simulink model "EcoSIM3_P2_C2"  (R2014b)
settings: Solver=ode1  SolverMode=SingleTasking  StartTime=0.0  StopTime=inf  FixedStep=0.01  RelTol=1e-3
PostLoadFcn:
  | %, if any(exist('dsrtsu_mdlpostloadfcn', 'file') == [2, 3, 6]), try dsrtsu_mdlpostloadfcn('Execute', bdroot); catch fprintf('Error in PostLoadFcn (dsrtsu_mdlpostloadfcn) for model "%s":\n %s\n', bdroot, lasterr); end, end,
InitFcn:
  | tic
  | %Startup_EcoSIM
values from neighbouring files (symbols this model uses):
  EngPwr = [0 5	10	15	20	25	30	35	40	45	50	55	60	65	70	75	80	85	90	95	100	105	110	115]    [Series_Maps.m]
  EngSpd = [0 477.4645 954.929 1909.858 2864.787 3819.716 4774.645 5729.574 6684.503]    [Series_Maps.m]
  EngTrq = [0	0	0	0	0	0	0	0	0	0	0	0	0	0	0	0	0	0	0	0	0	0	0	0 ... (first row only)    [Series_Maps.m]
  Power = [0 5 10 15 20 25 30]    [Series_Maps.m]
  Torque = [-50,-40,-30,-25,-20,-15,-10,-8,-6,-4,-2,0]    [Series_Maps.m]
undefined symbols (not defined in the file or in its folder): canChannel, Controls, DriveCycles, Driver, EM_EFF_MAP, EM_PwrLoss_MAP, Glbl, Plants, Veh_Dynamics
libraries: canmsglib x100, canlib x87, fl_lib x78, simulink x59, nesl_utility x40, sdl_lib x17, dspsigops x5, dspswit3 x3, dspstat3 x2, commnoisgen2 x1, dspfdesign x1
(part 7 of 15)

== system EcoSIM3_P2_C2/Supervisory Controller/Supervisory_IO/VNT Vector/Electrical Tx ==
  Electrical Tx : Inport
  Bus Creator : BusCreator  Inputs=2
  Bus Selector : BusSelector  OutputSignals=PON,chga_wake
  tag scope: VNT_Electrical_FromMABx=global
  wires:
  Bus Creator/1 -> [VNT_Electrical_FromMABx]  "Supervisory_Electrical_Out"
  Bus Selector/2 -> Bus Creator/2  "<chga_wake>"
  Bus Selector/1 -> Bus Creator/1  "<PON>"
  Electrical Tx/1 -> Bus Selector/1

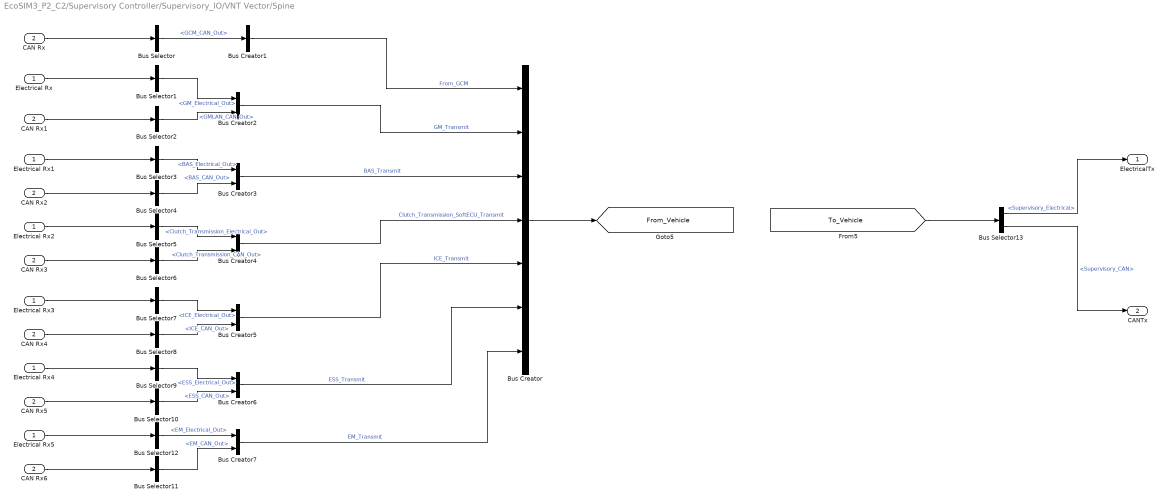
== system EcoSIM3_P2_C2/Supervisory Controller/Supervisory_IO/VNT Vector/Spine ==
  Electrical Rx : Inport
  CAN Rx : Inport  Port=2
  Bus Creator : BusCreator  Inputs=7
  Bus Creator1 : BusCreator  Inputs=1
  Bus Creator{2..7} (6 alike) : BusCreator  Inputs=2
  Bus Selector : BusSelector  OutputSignals=GCM_CAN_Out
  Bus Selector1 : BusSelector  OutputSignals=GM_Electrical_Out
  Bus Selector10 : BusSelector  OutputSignals=ESS_CAN_Out
  Bus Selector11 : BusSelector  OutputSignals=EM_CAN_Out
  Bus Selector12 : BusSelector  OutputSignals=EM_Electrical_Out
  Bus Selector13 : BusSelector  OutputSignals=Supervisory_Electrical,Supervisory_CAN
  Bus Selector2 : BusSelector  OutputSignals=GMLAN_CAN_Out
  Bus Selector3 : BusSelector  OutputSignals=BAS_Electrical_Out
  Bus Selector4 : BusSelector  OutputSignals=BAS_CAN_Out
  Bus Selector5 : BusSelector  OutputSignals=Clutch_Transmission_Electrical_Out
  Bus Selector6 : BusSelector  OutputSignals=Clutch_Transmission_CAN_Out
  Bus Selector7 : BusSelector  OutputSignals=ICE_Electrical_Out
  Bus Selector8 : BusSelector  OutputSignals=ICE_CAN_Out
  Bus Selector9 : BusSelector  OutputSignals=ESS_Electrical_Out
  CAN Rx{1..6} (6 alike) : InportShadow  Port=2
  Electrical Rx{1..5} (5 alike) : InportShadow
  ElectricalTx : Outport
  CANTx : Outport  Port=2
  tag scope: From_Vehicle=global
  wires:
  [To_Vehicle] -> Bus Selector13/1
  Bus Creator/1 -> [From_Vehicle]
  CAN Rx/1 -> Bus Selector/1
  Electrical Rx/1 -> Bus Selector1/1
  Bus Selector/1 -> Bus Creator1/1  "<GCM_CAN_Out>"
  Bus Creator1/1 -> Bus Creator/1  "From_GCM"
  CAN Rx1/1 -> Bus Selector2/1
  Bus Selector1/1 -> Bus Creator2/1  "<GM_Electrical_Out>"
  Bus Selector2/1 -> Bus Creator2/2  "<GMLAN_CAN_Out>"
  Bus Creator2/1 -> Bus Creator/2  "GM_Transmit"
  Electrical Rx1/1 -> Bus Selector3/1
  CAN Rx2/1 -> Bus Selector4/1
  Bus Selector3/1 -> Bus Creator3/1  "<BAS_Electrical_Out>"
  Bus Selector4/1 -> Bus Creator3/2  "<BAS_CAN_Out>"
  Bus Creator3/1 -> Bus Creator/3  "BAS_Transmit"
  Electrical Rx2/1 -> Bus Selector5/1
  CAN Rx3/1 -> Bus Selector6/1
  Bus Selector5/1 -> Bus Creator4/1  "<Clutch_Transmission_Electrical_Out>"
  Bus Selector6/1 -> Bus Creator4/2  "<Clutch_Transmission_CAN_Out>"
  Bus Creator4/1 -> Bus Creator/4  "Clutch_Transmission_SoftECU_Transmit"
  Electrical Rx3/1 -> Bus Selector7/1
  CAN Rx4/1 -> Bus Selector8/1
  Bus Selector7/1 -> Bus Creator5/1  "<ICE_Electrical_Out>"
  Bus Selector8/1 -> Bus Creator5/2  "<ICE_CAN_Out>"
  Bus Creator5/1 -> Bus Creator/5  "ICE_Transmit"
  Electrical Rx4/1 -> Bus Selector9/1
  CAN Rx5/1 -> Bus Selector10/1
  Bus Selector9/1 -> Bus Creator6/1  "<ESS_Electrical_Out>"
  Bus Selector10/1 -> Bus Creator6/2  "<ESS_CAN_Out>"
  Bus Creator6/1 -> Bus Creator/6  "ESS_Transmit"
  Electrical Rx5/1 -> Bus Selector12/1
  CAN Rx6/1 -> Bus Selector11/1
  Bus Selector12/1 -> Bus Creator7/1  "<EM_Electrical_Out>"
  Bus Selector11/1 -> Bus Creator7/2  "<EM_CAN_Out>"
  Bus Creator7/1 -> Bus Creator/7  "EM_Transmit"
  Bus Selector13/1 -> ElectricalTx/1  "<Supervisory_Electrical>"
  Bus Selector13/2 -> CANTx/1  "<Supervisory_CAN>"

== system EcoSIM3_P2_C2/Powertrain/BAS Motor/ Compnent Model/Sensors/Sensor lag ==
  i : Inport
  1st Order LPF of 1ms in Discrete Form : DiscreteTransferFcn  Numerator=[0.6321]  Denominator=[1 -0.3679]
  o : Outport
  wires:
  i/1 -> 1st Order LPF of 1ms in Discrete Form/1
  1st Order LPF of 1ms in Discrete Form/1 -> o/1

== system EcoSIM3_P2_C2/Powertrain/BAS Motor/ Compnent Model/Sensors/Sensor lag1 ==
  i : Inport
  1st Order LPF of 1ms in Discrete Form : DiscreteTransferFcn  Numerator=[0.6321]  Denominator=[1 -0.3679]
  o : Outport
  wires:
  1st Order LPF of 1ms in Discrete Form/1 -> o/1
  i/1 -> 1st Order LPF of 1ms in Discrete Form/1

== system EcoSIM3_P2_C2/Powertrain/BAS Motor/Soft ECU/Algorithm/BAS_Stateflow ==
  note: Notes:
      | 1. Mode Request is similar to Inverter Enable / Disable (to be received from the supervisory controller)
      | 2. Motor Fault is detected by a fault appearing at any of the phases of the motor (other faults can be incorporated in the Fault Subsystem)
  ModeRequest : Inport
  TorqueLimit : Inport  Port=2
  TorqueCommand : Inport  Port=3
  MotorSpeed : Inport  Port=4
  PowerUp : Inport  Port=5
  Speed_cmd : Inport  Port=6
  BAS SoftECU : Stateflow chart  TreatAsAtomicUnit=on
  Bus Creator : BusCreator  Inputs=6
  Bus Selector : BusSelector  OutputSignals=Fault_U,Fault_V,Fault_W
  Bus Selector2 : BusSelector  OutputSignals=Motor_MaxSpeed,POST_Fault
  Constant : Constant  Value=Plants.Belt.GR  SampleTime=0.01
  Contactor_Status : Constant
  Display : Display
  EEPROM Parameters : Subsystem
  Faults : Subsystem
  Gain : Gain  Gain=-1
  Ground : Ground
  Logical Operator : Logic  AllPortsSameDT=off  OutDataTypeStr=boolean
  Multiport Switch : MultiPortSwitch  DataPortOrder=Zero-based contiguous  SampleTime=0.01
  Saturation Dynamic : simulink/Discontinuities/Saturation Dynamic  OutMin=[]  OutMax=[]  OutDataTypeStr=Inherit: Same as second input  OutDataType=fixdt(1, 16)  OutScaling=2^-10  DoSatur=off
  Subsystem : Subsystem
  BAS_Torque_Command_Nm : Outport
  BAS_CAN_Out : Outport  Port=2
  wires:
  EEPROM Parameters/1(EEPROM param) -> Bus Selector2/1
  Bus Selector2/2 -> BAS SoftECU/5(POST_Fault)  "<POST_Fault>"
  Contactor_Status/1 -> Logical Operator/2  "batt_mainc_stat"
  Logical Operator/1 -> BAS SoftECU/1(Power_up)  "Power_up"
  Faults/1(MotorFault) -> BAS SoftECU/2(MotorFault)
  ModeRequest/1 -> Multiport Switch/1, BAS SoftECU/3(ModeRequest)
  Bus Selector2/1 -> BAS SoftECU/4(MotorMaxSpeed)  "<Motor_MaxSpeed>"
  Gain/1 -> Saturation Dynamic/3
  TorqueLimit/1 -> Saturation Dynamic/1, Gain/1
  TorqueCommand/1 -> Saturation Dynamic/2
  MotorSpeed/1 -> Subsystem/2(Speed_feedback_rad_per_s), BAS SoftECU/7(MotorSpeed)
  BAS SoftECU/1(Commanded_Torque) -> Multiport Switch/3, Bus Creator/1
  BAS SoftECU/2(InverterStatusMode) -> Bus Creator/2  "BAS_Status_Mode"
  Bus Creator/1 -> BAS_CAN_Out/1  "BAS CAN Out"
  Faults/2(CAN) -> Bus Selector/1
  Bus Selector/3 -> Bus Creator/6  "<Fault_W>"
  Bus Selector/2 -> Bus Creator/5  "<Fault_V>"
  Bus Selector/1 -> Bus Creator/4  "<Fault_U>"
  BAS SoftECU/3(FaultState) -> Bus Creator/3  "BAS_Fault_Status"
  PowerUp/1 -> Logical Operator/1
  Constant/1 -> BAS SoftECU/8(BeltRatio), Display/1
  Multiport Switch/1 -> BAS_Torque_Command_Nm/1
  Speed_cmd/1 -> BAS SoftECU/9(Speed_Command)
  BAS SoftECU/4(Commanded_Speed) -> Subsystem/1(Speed_command_rpm)
  Ground/1 -> Multiport Switch/2
  Subsystem/1("Torque_command_Nm ") -> Multiport Switch/4
  Saturation Dynamic/1 -> BAS SoftECU/6(Torque_Command)

== system EcoSIM3_P2_C2/Powertrain/Electric Motor / Component Model/Plant/EM_Thermal_Model ==
  note: Instead of a heat source, add convection to the water
  note: A hotspot that will be the thermally weakest point
  note: Assume coolant out temp is same as motor temp
  EM_Power_Loss : Inport
  Conductive Heat Transfer : fl_lib/Thermal/Thermal Elements/Conductive Heat Transfer  area=4 cm^2  thickness=0.1 cm  th_cond=401 W/(m*K)  Q_specify=off  Q_priority=High  Q=0 J/s  T_specify=off  T_priority=High  T=0 K
  Constant1 : Constant  Value=293
  Convection to air : fl_lib/Thermal/Thermal Elements/Convective Heat Transfer  area=1111 cm^2  heat_tr_coeff=10 W/(m^2 * K)  Q_specify=off  Q_priority=High  Q=0 J/s  T_specify=off  T_priority=High  T=0 K
  EM_Over_Temp_Fault : Subsystem
  Gain : Gain  Gain=0.05
  Gain1 : Gain  Gain=0.95
  Heat Dissipated through coolant : Subsystem
  Heat absorbed by coolant : fl_lib/Thermal/Thermal Sources/Ideal Heat Flow Source
  Hotspot Heat : fl_lib/Thermal/Thermal Sources/Ideal Heat Flow Source
  Hotspot Thermal mass : fl_lib/Thermal/Thermal Elements/Thermal Mass  mass=0.1 kg  sp_heat=447 J/kg/K  Q_specify=off  Q_priority=High  Q=0 J/s  T_specify=off  T_priority=High  T=300 K
  Hotspot temp in °C : Scope
      settings: SaveName=ScopeData2
  Ideal Temperature Source : fl_lib/Thermal/Thermal Sources/Ideal Temperature Source
  Memory : Memory  X0=293
  Memory1 : Memory  X0=25
  Motor Heat Loss : fl_lib/Thermal/Thermal Sources/Ideal Heat Flow Source
  Motor Thermal Mass : fl_lib/Thermal/Thermal Elements/Thermal Mass  mass=35 kg  sp_heat=447 J/kg/K  Q_specify=off  Q_priority=High  Q=0 J/s  T_specify=off  T_priority=High  T=300 K
  Simulink-PS Converter : nesl_utility/Simulink-PS Converter  PhysicalDomain=network_engine_domain  SubClassName=ps_input  LeftPortType=input  RightPortType=output  PseudoPeriodic=off  Frequencies=[]  NoiseDistribution=none  NoiseParameters=[]  Unit=J/s  AffineConversion=off  InputFiltering=off  SimscapeFilterOrder=1  InputFilterTimeConstant=0.001  UdotUserProvided=1
  Simulink-PS Converter1 : nesl_utility/Simulink-PS Converter  PhysicalDomain=network_engine_domain  SubClassName=ps_input  LeftPortType=input  RightPortType=output  PseudoPeriodic=off  Frequencies=[]  NoiseDistribution=none  NoiseParameters=[]  Unit=J/s  AffineConversion=off  InputFiltering=off  SimscapeFilterOrder=1  InputFilterTimeConstant=0.001  UdotUserProvided=1
  Simulink-PS Converter2 : nesl_utility/Simulink-PS Converter  PhysicalDomain=network_engine_domain  SubClassName=ps_input  LeftPortType=input  RightPortType=output  PseudoPeriodic=off  Frequencies=[]  NoiseDistribution=none  NoiseParameters=[]  Unit=K  AffineConversion=off  InputFiltering=off  SimscapeFilterOrder=1  InputFilterTimeConstant=0.001  UdotUserProvided=1
  Solver Configuration : nesl_utility/Solver Configuration  PhysicalDomain=network_engine_domain  SubClassName=solver  LeftPortType=input  RightPortType=generic  Accelerate=off  Tones=[]  Harmonics=[]  SimulateNoise=off  Profile=off  UseLocalSampling=off  EnableSwitchedLinearOptims=on  FrequencyDomain=off  UseCCode=off  RelTol=0.001  AbsTol=1e-06  MinStep=1e-09  ToWorkspace=off  DoDC=off  ResidualTolerance=1e-09  UseLocalSolver=on  LocalSolverChoice=NE_BACKWARD_EULER_ADVANCER  LocalSolverSampleTime=0.01  DoFixedCost=off  MaxNonlinIter=3  MaxModeIter=2  LinearAlgebra=Sparse  DelaysMemoryBudget=1024  AutomaticFiltering=on  FilteringTimeConstant=0.001
  Temp Hotspot : Subsystem
  Temp Motor : Subsystem
  Thermal Reference{,2..4} (4 alike) : fl_lib/Thermal/Thermal Elements/Thermal Reference
  Out1 : Outport
  wires:
  Constant1/1 -> Simulink-PS Converter2/1
  Temp Hotspot/1(Temp C) -> Hotspot temp in °C/1  "EM_hotspot_Temperature_degC"
  Temp Motor/1(Temp K) -> Memory/1
  EM_Over_Temp_Fault/1(Out1) -> Out1/1  "EM_Temperature_degC"
  Memory/1 -> Heat Dissipated through coolant/1(Coolant Out Temp)
  EM_Power_Loss/1 -> Gain/1, Gain1/1  "EM_Power_loss_W"
  Gain/1 -> Simulink-PS Converter/1
  Gain1/1 -> Simulink-PS Converter1/1
  Temp Motor/2(Temp C) -> Memory1/1  "EM_Temperature_degC"
  Memory1/1 -> EM_Over_Temp_Fault/1(In1)  "EM_Temperature_degC"
  connections:
  Simulink-PS Converter2/RConn1 -- Ideal Temperature Source/RConn1
  Heat Dissipated through coolant/RConn1 -- Heat absorbed by coolant/RConn1
  Convection to air/RConn1 -- Ideal Temperature Source/LConn1
  Thermal Reference4/LConn1 -- Hotspot Heat/RConn2
  Simulink-PS Converter1/RConn1 -- Hotspot Heat/RConn1
  Thermal Reference/LConn1 -- Motor Heat Loss/RConn2
  Thermal Reference2/LConn1 -- Ideal Temperature Source/RConn2
  Thermal Reference3/LConn1 -- Heat absorbed by coolant/RConn2
  Motor Heat Loss/RConn1 -- Simulink-PS Converter/RConn1 -- Solver Configuration/RConn1
  Convection to air/LConn1 -- Temp Motor/LConn1 -- Conductive Heat Transfer/RConn1 -- Motor Thermal Mass/LConn1 -- Heat absorbed by coolant/LConn1 -- Motor Heat Loss/LConn1
  Conductive Heat Transfer/LConn1 -- Hotspot Thermal mass/LConn1 -- Temp Hotspot/LConn1 -- Hotspot Heat/LConn1

== system EcoSIM3_P2_C2/Powertrain/Electric Motor / Component Model/Sensors/Fault Insertation ==
  In1 : Inport
  Additional_Torque_Nm_Default : Constant  Value=0
  Gain : Gain  Gain=.3
  Ideal Torque Source1 : fl_lib/Mechanical/Mechanical Sources/Ideal Torque Source
  Mechanical Rotational Reference2 : fl_lib/Mechanical/Rotational Elements/Mechanical Rotational Reference
  OverTorque_Trigger : Switch  Criteria=u2 > Threshold  Threshold=0.5
  Simulink-PS Converter1 : nesl_utility/Simulink-PS Converter  PhysicalDomain=network_engine_domain  SubClassName=ps_input  LeftPortType=input  RightPortType=output  PseudoPeriodic=off  Frequencies=[]  NoiseDistribution=none  NoiseParameters=[]  Unit=1  AffineConversion=off  InputFiltering=off  SimscapeFilterOrder=1  InputFilterTimeConstant=0.001  UdotUserProvided=1
  Conn1 : PMIOPort  Port=1  Side=Right
  wires:
  [EM_OverTorque_Trigger] -> OverTorque_Trigger/2
  Additional_Torque_Nm_Default/1 -> OverTorque_Trigger/3
  OverTorque_Trigger/1 -> Simulink-PS Converter1/1
  In1/1 -> Gain/1
  Gain/1 -> OverTorque_Trigger/1
  connections:
  Simulink-PS Converter1/RConn1 -- Ideal Torque Source1/RConn1
  Ideal Torque Source1/RConn2 -- Mechanical Rotational Reference2/LConn1
  Ideal Torque Source1/LConn1 -- Conn1/RConn1

== system EcoSIM3_P2_C2/Powertrain/Electric Motor / Component Model/Sensors/Sensor lag ==
  i : Inport
  1st Order LPF of 1ms in Discrete Form : DiscreteTransferFcn  Numerator=[0.6321]  Denominator=[1 -0.3679]
  o : Outport
  wires:
  i/1 -> 1st Order LPF of 1ms in Discrete Form/1
  1st Order LPF of 1ms in Discrete Form/1 -> o/1

== system EcoSIM3_P2_C2/Powertrain/Electric Motor / Component Model/Sensors/Sensor lag1 ==
  i : Inport
  1st Order LPF of 1ms in Discrete Form : DiscreteTransferFcn  Numerator=[0.6321]  Denominator=[1 -0.3679]
  o : Outport
  wires:
  i/1 -> 1st Order LPF of 1ms in Discrete Form/1
  1st Order LPF of 1ms in Discrete Form/1 -> o/1

== system EcoSIM3_P2_C2/Powertrain/Electric Motor / Component Model/Sensors/Sensors ==
  note: Sensor Model: Place where we add Corrupter
  Bus Creator : BusCreator  Inputs=2
  Ideal Rotational Motion Sensor : fl_lib/Mechanical/Mechanical Sensors/Ideal Rotational Motion Sensor  offset=0 rad
  Ideal Torque Sensor : fl_lib/Mechanical/Mechanical Sensors/Ideal Torque Sensor
  Mechanical Rotational Reference1 : fl_lib/Mechanical/Rotational Elements/Mechanical Rotational Reference
  PS-Simulink Converter : nesl_utility/PS-Simulink Converter  PhysicalDomain=network_engine_domain  SubClassName=ps_output  LeftPortType=input  RightPortType=output  PseudoPeriodic=off  Frequencies=[]  Unit=1  AffineConversion=off
  PS-Simulink Converter1 : nesl_utility/PS-Simulink Converter  PhysicalDomain=network_engine_domain  SubClassName=ps_output  LeftPortType=input  RightPortType=output  PseudoPeriodic=off  Frequencies=[]  Unit=1  AffineConversion=off
  Sensor lag : Subsystem
  Sensor lag1 : Subsystem
  Shaft : PMIOPort  Port=1  Side=Left
  To_Plants : PMIOPort  Port=2  Side=Right
  EM_Shaft_out : Outport
  wires:
  Sensor lag/1(o) -> Bus Creator/1  "EM_Speed_produced_rad_per_s"
  Sensor lag1/1(o) -> Bus Creator/2  "EM_Torque_Produced_Nm"
  Bus Creator/1 -> EM_Shaft_out/1  "EM_Shaft"
  PS-Simulink Converter/1 -> Sensor lag/1(i)  "EM_Speed_produced_rad_per_s"
  PS-Simulink Converter1/1 -> Sensor lag1/1(i)  "EM_Torque_Produced_Nm"
  connections:
  Ideal Torque Sensor/LConn1 -- Shaft/RConn1 -- Ideal Rotational Motion Sensor/LConn1
  Ideal Rotational Motion Sensor/RConn1 -- Mechanical Rotational Reference1/LConn1
  PS-Simulink Converter/LConn1 -- Ideal Rotational Motion Sensor/RConn2
  PS-Simulink Converter1/LConn1 -- Ideal Torque Sensor/RConn2
  Ideal Torque Sensor/RConn1 -- To_Plants/RConn1

== system EcoSIM3_P2_C2/Powertrain/Electric Motor /Soft ECU/Algorithm/Normal Operation ==
  note: These signals are supposed to be
      |  coming in through CAN
  SignalIn : Inport
  Ignition Switch : Inport  Port=2
  FaultTrigger : Inport  Port=3
  Sensors : Inport  Port=4
  Enable : EnablePort  StatesWhenEnabling=reset
  Bus Selector : BusSelector  OutputSignals=Motor_MaxSpeed
  Bus Selector1 : BusSelector  OutputSignals=EM_CAN_Messages.EM_CAN.M192_Command_Message.Rotation_Direction,EM_CAN_Messages.EM_CAN.M192_Command_Message.Torque_Command,ESS_CAN_Out.BCM_Status.bcm_mainc_stat,EM_CAN_Messages.EM_CAN.M192_Command_Message.Inverter_Enable
  Bus Selector2 : BusSelector  OutputSignals=Motor_Speed,InternalMotorError
  Bus Selector3 : BusSelector  OutputSignals=GMLAN_CAN_Out.PPEI_Platform_General_Status.SysPwrMd
  Bus Selector4 : BusSelector  OutputSignals=EM_torque_cmd_value,EM_torque_cmd_trigger
  EEPROM Parameters1 : Subsystem
  Normal_Operation : Stateflow chart  TreatAsAtomicUnit=on
  Switch : Switch  Criteria=u2 > Threshold  Threshold=0.5
  Commanded_Torque : Outport
  RUN_Fault : Outport  Port=2
  ShutdownRequest : Outport  Port=3  OutputWhenDisabled=reset  InitialOutput=0
  wires:
  Normal_Operation/2(RUN_Fault) -> RUN_Fault/1
  Bus Selector1/1 -> Normal_Operation/3(Rotation_Direction)  "<Rotation_Direction>"
  Bus Selector1/2 -> Normal_Operation/4(Torque_Command)  "<Torque_Command>"
  SignalIn/1 -> Bus Selector1/1
  Bus Selector/1 -> Normal_Operation/8(Motor_MaxSpeed)  "<Motor_MaxSpeed>"
  Sensors/1 -> Bus Selector2/1
  Bus Selector2/1 -> Normal_Operation/1(Motor_Speed)  "<Motor_Speed>"
  Bus Selector2/2 -> Normal_Operation/2(InternalMotorError)  "<InternalMotorError>"
  Normal_Operation/1(Commanded_Torque) -> Switch/3
  EEPROM Parameters1/1(EEPROM param) -> Bus Selector/1
  Bus Selector1/3 -> Normal_Operation/5(batt_mainc_stat)  "<bcm_mainc_stat>"
  Ignition Switch/1 -> Bus Selector3/1
  Bus Selector3/1 -> Normal_Operation/7(IgnitionKeySw)  "<SysPwrMd>"
  Normal_Operation/3(ShutdownRequest) -> ShutdownRequest/1
  Bus Selector1/4 -> Normal_Operation/6(Inverter_Enable)  "<Inverter_Enable>"
  Switch/1 -> Commanded_Torque/1  "Commanded_Torque"
  FaultTrigger/1 -> Bus Selector4/1
  Bus Selector4/2 -> Switch/2  "<EM_torque_cmd_trigger>"
  Bus Selector4/1 -> Switch/1  "<EM_torque_cmd_value>"

== system EcoSIM3_P2_C2/Powertrain/Electric Motor /Soft ECU/Algorithm/Rinehart Documentation ==

== system EcoSIM3_P2_C2/Powertrain/Electric Motor /Soft ECU/Algorithm/Startup_Shutdown ==
  SignalIn : Inport
  Ignition Switch : Inport  Port=2
  RUN_Fault : Inport  Port=3
  ShutDownRequest : Inport  Port=4
  Bus Selector : BusSelector  OutputSignals=EM_CAN_Messages.EM_Electrical.EM_Powerup,EM_Sensors.InternalMotorError,ESS_CAN_Out.BCM_Status.bcm_mainc_stat,EM_CAN_Messages.EM_CAN.M192_Command_Message.Inverter_Enable
  Bus Selector1 : BusSelector  OutputSignals=KeySwMode,POST_Fault
  Bus Selector2 : BusSelector  OutputSignals=GMLAN_CAN_Out.PPEI_Platform_General_Status.SysPwrMd
  Bus Selector3 : BusSelector  Commented=on  OutputSignals=EM_Powerup
  Display : Display
  Display1 : Display
  EEPROM Parameters : Subsystem
  From : From  Commented=on  GotoTag=Powerups  TagVisibility=global
  Memory : Memory
  Startup-Shutdown : Stateflow chart  TreatAsAtomicUnit=on
  VSM_Mode : Outport
  Inverter_Enable_Lockout : Outport  Port=2
  Inverter_Status : Outport  Port=3
  POST_Fault : Outport  Port=4
  wires:
  Startup-Shutdown/1(VSM_Mode) -> VSM_Mode/1
  Startup-Shutdown/2(Inverter_Enable_Lockout) -> Display1/1, Inverter_Enable_Lockout/1  "Inverter_Enable_Lockout"
  RUN_Fault/1 -> Startup-Shutdown/6(RUN_Fault)
  ShutDownRequest/1 -> Memory/1
  Bus Selector/2 -> Startup-Shutdown/2(InternalMotorError)  "<InternalMotorError>"
  SignalIn/1 -> Bus Selector/1
  EEPROM Parameters/1(EEPROM param) -> Bus Selector1/1
  Bus Selector1/1 -> Startup-Shutdown/8(KeySwMode)  "<KeySwMode>"
  Bus Selector1/2 -> POST_Fault/1, Startup-Shutdown/9(POST_Fault)  "<POST_Fault>"
  Bus Selector/3 -> Startup-Shutdown/3(batt_mainc_stat)  "<bcm_mainc_stat>"
  Bus Selector/4 -> Display/1, Startup-Shutdown/4(Inverter_Enable)  "<Inverter_Enable>"
  Startup-Shutdown/3(Inverter_Status) -> Inverter_Status/1
  Ignition Switch/1 -> Bus Selector2/1
  Bus Selector2/1 -> Startup-Shutdown/5(IgnitionKeySw)  "<SysPwrMd>"
  Memory/1 -> Startup-Shutdown/7(ShutdownRequest)
  Bus Selector/1 -> Startup-Shutdown/1(Power_up)  "<EM_Powerup>"

== system EcoSIM3_P2_C2/Powertrain/Electric Motor /Soft ECU/Algorithm/Temperature Values Dummy ==
  FromPlant : Inport
  Bus Creator : BusCreator  Inputs=6
  Control_Board_Temperature : Constant  Value=25
  ESS_Over_Temp_Fault : Subsystem
  Gain : Gain
  Gate_Driver_Board : Constant  Value=25
  Module_A : Constant  Value=25
  Module_B : Constant  Value=25
  Module_C : Constant  Value=25
  TempValues : Outport
  wires:
  ESS_Over_Temp_Fault/1(Out1) -> Bus Creator/1  "Module_A"
  Bus Creator/1 -> TempValues/1
  Module_B/1 -> Bus Creator/2  "Module_B"
  Module_C/1 -> Bus Creator/3  "Module_C"
  Gate_Driver_Board/1 -> Bus Creator/4  "Gate_Driver_Board"
  Control_Board_Temperature/1 -> Bus Creator/5  "Control_Board_Temperature"
  FromPlant/1 -> Gain/1
  Gain/1 -> Bus Creator/6  "Motor_Temperature"
  Module_A/1 -> ESS_Over_Temp_Fault/1(In1)

== system EcoSIM3_P2_C2/Powertrain/Electrical Storage System/ ESS Model/Plant/Electrical Plant Model ==
  P_in [W] : Inport
  Batt_Temp [C] : Inport  Port=2
  Current Calculation (Per Cell) : Subsystem
  Heat Calculation : Subsystem
  Memory1 : Memory  X0=300
  OCV Estimation : Subsystem
  "Resistance Estimation (Per Cell) " : Subsystem
  SOC Estimation (Per Cell) : Subsystem
  Terminal Voltage Calculation : Subsystem
  Batt_Current [A] : Outport
  Batt_SOC [%] : Outport  Port=2
  Batt_volt [V] : Outport  Port=3
  Batt_Heat [W] : Outport  Port=4
  Batt_volt_1 [V] : Outport  Port=5
  wires:
  P_in [W]/1 -> SOC Estimation (Per Cell)/1(P_in [W]), Current Calculation (Per Cell)/1(P_in [W])
  Terminal Voltage Calculation/1(Batt_Volt [V]) -> Batt_volt [V]/1, Memory1/1
  Current Calculation (Per Cell)/2(Cell_Current [A]) -> "Resistance Estimation (Per Cell) "/1(Cell_Current [A]), Heat Calculation/1(Cell_Current [A]), Terminal Voltage Calculation/3(Cell_Current [A]), OCV Estimation/2(Cell_Current [A])
  SOC Estimation (Per Cell)/1(SOC [%]) -> "Resistance Estimation (Per Cell) "/3(SOC [%]), Batt_SOC [%]/1, OCV Estimation/1(SOC [%])
  OCV Estimation/1(OCV [V]) -> Terminal Voltage Calculation/2(OCV [V])
  Current Calculation (Per Cell)/1(Batt_Current [A]) -> Batt_Current [A]/1
  Heat Calculation/1(Batt_Heat [W]) -> Batt_Heat [W]/1
  "Resistance Estimation (Per Cell) "/1(R_cell [Ohms]) -> Terminal Voltage Calculation/1(R_cell [Ohms]), Heat Calculation/2(R_cell [Ohms])
  Memory1/1 -> Batt_volt_1 [V]/1, Current Calculation (Per Cell)/2(Batt_volt [V])
  Batt_Temp [C]/1 -> "Resistance Estimation (Per Cell) "/2(Cell_Temp [C])

== system EcoSIM3_P2_C2/Powertrain/Electrical Storage System/ ESS Model/Plant/Power Calculation ==
  Input_Crnt [A] : Inport
  Batt_volt_1 [V] : Inport  Port=2
  Component_Power_Watts : Inport  Port=3
  Avg Power Calculation : Subsystem
  Integrator1 : Integrator
  P_in [W] : Outport
  Batt_Electrical_Energy : Outport  Port=2
  Batt_Electrical_Energy_Net : Outport  Port=3
  wires:
  Avg Power Calculation/1(P_in [W]) -> Batt_Electrical_Energy/1, Integrator1/1, P_in [W]/1  "Batt_Electrical_Energy"
  Input_Crnt [A]/1 -> Avg Power Calculation/1(Input_Crnt [A])
  Batt_volt_1 [V]/1 -> Avg Power Calculation/2(Batt_volt_1 [V])
  Integrator1/1 -> Batt_Electrical_Energy_Net/1  "Batt_Electrical_Energy_Net"
  Component_Power_Watts/1 -> Avg Power Calculation/3(Component_Power_Watts)

== system EcoSIM3_P2_C2/Powertrain/Electrical Storage System/ ESS Model/Plant/Thermal Model ==
  note: 1/7
  note: 273+30
  Batt_Heat [W] : Inport
  Constant : Constant  Value=Plants.ESS.Mdl.Plant.Therm_Mdl.T_amb
  Constant5 : Constant  Value=273
  EM_Over_Temp_Fault : Subsystem
  Fcn2 : Fcn  Expr=u/19395
  Fcn3 : Fcn  Expr=u/(193.52*19395)
  Heat input for pack1 : Gain  Gain=1/Plants.ESS.Mdl.Plant.Therm_Mdl.M
  Integrator : Integrator  InitialConditionSource=external
  Subtract : Sum  Inputs=+-
  Subtract3 : Sum  Inputs=-+
  Subtract4 : Sum  Inputs=+-
  T_ambient : Constant  Value=Plants.ESS.Mdl.Plant.Therm_Mdl.T_amb
  Batt_Temp [C] : Outport
  wires:
  Batt_Heat [W]/1 -> Heat input for pack1/1
  Integrator/1 -> Subtract/1, Subtract4/1  "T_B"
  Subtract3/1 -> Integrator/1  "T_B_dot"
  T_ambient/1 -> Subtract/2
  Subtract/1 -> Fcn3/1
  Fcn2/1 -> Subtract3/2
  Constant/1 -> Integrator/2
  Constant5/1 -> Subtract4/2
  EM_Over_Temp_Fault/1(Out1) -> Batt_Temp [C]/1  "Batt_Temp_C"
  Heat input for pack1/1 -> Fcn2/1
  Fcn3/1 -> Subtract3/1
  Subtract4/1 -> EM_Over_Temp_Fault/1(In1)  "Batt_Temp_C"

== system EcoSIM3_P2_C2/Powertrain/Electrical Storage System/Soft ECU/Algorithm/A123 Documentation ==

== system EcoSIM3_P2_C2/Powertrain/Electrical Storage System/Soft ECU/Algorithm/A123 soft ECU ==
  From ECUs : Inport
  A123 BMS : Stateflow chart  TreatAsAtomicUnit=on
  Bus Creator : BusCreator  Inputs=11
  Bus Selector : BusSelector  OutputSignals=BMS_Powerup,hsc_bcm_enable,hsc_bcm_mainc_close,bcm_cell_tmax,hsc_bcm_epo,hsc_bcm_leakage_ena,chga_wake
  Bus Selector1 : BusSelector  OutputSignals=GMLAN_CAN_Out.PPEI_Platform_General_Status.SysPwrMd
  Bus Selector2 : BusSelector  OutputSignals=bcm_alarm_type,bcm_alarm_trigger
  Constant : Constant  Value=65
  Constant1 : Constant  Value=-40
  Constant2 : Constant  Value=0
  Memory{,1..10} (11 alike) : Memory
  Switch : Switch  Criteria=u2 > Threshold  Threshold=0.5
  To ECUs : Outport
  wires:
  From ECUs/1 -> Bus Selector/1
  Bus Selector/2 -> A123 BMS/2(hsc_bcm_enable)  "<hsc_bcm_enable>"
  Bus Selector/3 -> A123 BMS/3(hsc_bcm_mainc_close)  "<hsc_bcm_mainc_close>"
  Constant/1 -> A123 BMS/5(bcm_cell_tmax)
  Constant1/1 -> A123 BMS/6(bcm_cell_tmin)
  Bus Selector/5 -> A123 BMS/7(hsc_bcm_epo)  "<hsc_bcm_epo>"
  Memory3/1 -> Bus Creator/4  "bcm_chgc_stat"
  Memory1/1 -> Bus Creator/3  "bcm_mainc_stat"
  Memory2/1 -> Bus Creator/5  "bcm_cpwr_cmd"
  Memory4/1 -> Bus Creator/2  "bcm_hvil_mon"
  Memory5/1 -> Bus Creator/6  "bcm_cpwr_mon"
  Memory/1 -> Bus Creator/1  "bcm_ready"
  Memory6/1 -> Bus Creator/7  "bcm_epo"
  Bus Creator/1 -> To ECUs/1
  Bus Selector/6 -> A123 BMS/8(hsc_bcm_leakage_ena)  "<hsc_bcm_leakage_ena>"
  [GM_Transmit] -> Bus Selector1/1
  Bus Selector1/1 -> A123 BMS/10(Veh_Start)  "<SysPwrMd>"
  A123 BMS/1(bcm_ready) -> Memory/1  "bcm_ready"
  A123 BMS/4(bcm_chgc_stat) -> Memory3/1  "bcm_chgc_stat"
  A123 BMS/7(bcm_epo) -> Memory6/1  "bcm_epo"
  A123 BMS/6(bcm_cpwr_mon) -> Memory5/1  "bcm_cpwr_mon"
  A123 BMS/5(bcm_cpwr_cmd) -> Memory2/1  "bcm_cpwr_cmd"
  A123 BMS/3(bcm_mainc_stat) -> Memory1/1  "bcm_mainc_stat"
  A123 BMS/2(bcm_hvil_mon) -> Memory4/1  "bcm_hvil_mon"
  Memory7/1 -> Bus Creator/8  "bcm_veh_mon"
  A123 BMS/8(bcm_veh_mon) -> Memory7/1
  Bus Selector/1 -> A123 BMS/1(PowerUp)  "<BMS_Powerup>"
  A123 BMS/9(chga_ena) -> Memory8/1
  Memory8/1 -> Bus Creator/9  "chga_ena"
  Bus Selector/7 -> A123 BMS/9(chga_wake)  "<chga_wake>"
  A123 BMS/10(bcm_on_plug) -> Memory9/1
  Memory9/1 -> Bus Creator/10  "bcm_on_plug"
  Bus Selector/4 -> A123 BMS/4(bcm_cell_temp)  "<bcm_cell_tmax>"
  Constant2/1 -> Switch/3
  Memory10/1 -> Bus Creator/11  "bcm_alarm"
  [BCM_Alarm_Trigger] -> Bus Selector2/1
  Bus Selector2/1 -> Switch/1  "<bcm_alarm_type>"
  Bus Selector2/2 -> Switch/2  "<bcm_alarm_trigger>"
  Switch/1 -> Memory10/1

== system EcoSIM3_P2_C2/Powertrain/Engine/ Component Model/Sensors/Sensor lag ==
  i : Inport
  1st Order LPF of 1ms in Discrete Form : DiscreteTransferFcn  Numerator=[0.6321]  Denominator=[1 -0.3679]
  o : Outport
  wires:
  i/1 -> 1st Order LPF of 1ms in Discrete Form/1
  1st Order LPF of 1ms in Discrete Form/1 -> o/1

== system EcoSIM3_P2_C2/Powertrain/Engine/ Component Model/Sensors/Sensor lag1 ==
  i : Inport
  1st Order LPF of 1ms in Discrete Form : DiscreteTransferFcn  Numerator=[0.6321]  Denominator=[1 -0.3679]
  o : Outport
  wires:
  i/1 -> 1st Order LPF of 1ms in Discrete Form/1
  1st Order LPF of 1ms in Discrete Form/1 -> o/1

== system EcoSIM3_P2_C2/Powertrain/Soft_ECUs_IO/From_Goto/Subsystem1/BAS_Relay ==
  In1 : Inport
  Constant6 : Constant
  Constant7 : Constant  Value=0
  Relay3 : Switch  Criteria=u2 > Threshold  Threshold=0.5
  Out1 : Outport
  wires:
  Constant6/1 -> Relay3/1
  Relay3/1 -> Out1/1  "BAS_Powerup"
  Constant7/1 -> Relay3/3
  In1/1 -> Relay3/2

== system EcoSIM3_P2_C2/Powertrain/Soft_ECUs_IO/From_Goto/Subsystem1/EM_Relay ==
  In1 : Inport
  Constant2 : Constant
  Constant3 : Constant  Value=0
  Relay1 : Switch  Criteria=u2 > Threshold  Threshold=0.5
  Out1 : Outport
  wires:
  Relay1/1 -> Out1/1  "EM_Powerup"
  Constant2/1 -> Relay1/1
  Constant3/1 -> Relay1/3
  In1/1 -> Relay1/2

== system EcoSIM3_P2_C2/Powertrain/Soft_ECUs_IO/From_Goto/Subsystem1/Engine_Relay ==
  In1 : Inport
  Constant4 : Constant
  Constant5 : Constant  Value=0
  Relay2 : Switch  Criteria=u2 > Threshold  Threshold=0.5
  Out1 : Outport
  wires:
  Relay2/1 -> Out1/1  "ICE_Powerup"
  Constant5/1 -> Relay2/3
  Constant4/1 -> Relay2/1
  In1/1 -> Relay2/2

== system EcoSIM3_P2_C2/Powertrain/Soft_ECUs_IO/VNT Kvaser/CANRx/BAS Receive ==
  Bus Creator12 : BusCreator  Inputs=1
  Bus Creator2 : BusCreator  Inputs=2
  CAN Receive : canlib/CAN Receive  BlockHandle=2745.0026  DeviceMenu=Kvaser Virtual 1 (Channel 1)  Device=Kvaser Virtual 1 (Channel 1)  ObjConstructor=canChannel('Kvaser', 'Virtual 1', 1)  EnableStandardIDsFilter=off  StandardIDs=102  EnableExtendedIDsFilter=off  ExtendedIDs=0  SampleTime=0.01  MsgsPerTimestep=1  StdIDsCombo=Allow only  ExtIDsCombo=Block all  InternalFilterUpdateStatus=on
  CAN Unpack : canmsglib/CAN Unpack  CANdbFile=C:\Users\EcoCAR_HIL\Documents\Khanna\EcoSIM3_P1_0_PHEV_TCU\Final_DBC\Engine_Transmission_BAS.dbc  MsgList=ECO_BAS_Receive_MSG102  MsgName=ECO_BAS_Receive_MSG102  MsgIDType=Standard (11-bit identifier)  MsgIdentifier=102  MsgLength=2  SignalInfo=BAS_Mode_Request$8$1$2$2$1$0$1$0$0$1$#BAS_Torque_Request_Nm$9$15$2$1$1$0$1.000000e-02$0$-1.638400e+02$1.638300e+02$#  NSignals=2  IDPort=off  TimestampPort=off  ErrorPort=off  RemotePort=off  LengthPort=off  StatusPort=off  StartBits=str2num('[int32(8);int32(9)]')  SignalSizes=str2num('[int32(1);int32(15)]')  ByteOrders=str2num('[int32(2);int32(2)]')  DataTypes=str2num('[int32(2);int32(1)]')  MultiplexTypes=str2num('[int32(1);int32(1)]')  MultiplexValues=str2num('[double(0);double(0)]')  Factors=str2num('[double(1);double(1.000000e-02)]')  Offsets=str2num('[double(0);double(0)]')  Minimums=str2num('[double(0);double(-1.638400e+02)]')  Maximums=str2num('[double(1);double(1.638300e+02)]')
      settings: DataFormat=CANdb specified signals
  Terminator6 : Terminator
  BAS_CAN : Outport
  wires:
  Bus Creator12/1 -> BAS_CAN/1  "BAS_CAN"
  Bus Creator2/1 -> Bus Creator12/1  "SetValues"
  CAN Receive/1 -> Terminator6/1
  CAN Unpack/1 -> Bus Creator2/1  "BAS_Mode_Request"
  CAN Unpack/2 -> Bus Creator2/2  "BAS_Torque_Request_Nm"
  CAN Receive/2 -> CAN Unpack/1

== system EcoSIM3_P2_C2/Powertrain/Soft_ECUs_IO/VNT Kvaser/CANRx/Brusa Receive ==
  Bus Creator4 : BusCreator  Inputs=2
  Ground : Ground
  Ground1 : Ground
  Brusa CAN : Outport
  wires:
  Bus Creator4/1 -> Brusa CAN/1  "Brusa_CAN"
  Ground/1 -> Bus Creator4/1  "Dummy1"
  Ground1/1 -> Bus Creator4/2  "Dummy2"

== system EcoSIM3_P2_C2/Powertrain/Soft_ECUs_IO/VNT Kvaser/CANRx/EM Receive ==
  Bus Creator : BusCreator  Inputs=1
  Bus Creator1 : BusCreator  Inputs=3
  CAN Receive1 : canlib/CAN Receive  BlockHandle=2767.0024  DeviceMenu=Kvaser Virtual 1 (Channel 2)  Device=Kvaser Virtual 1 (Channel 2)  ObjConstructor=canChannel('Kvaser', 'Virtual 1', 2)  EnableStandardIDsFilter=off  StandardIDs=192  EnableExtendedIDsFilter=off  ExtendedIDs=0  SampleTime=0.01  MsgsPerTimestep=1  StdIDsCombo=Allow only  ExtIDsCombo=Block all  InternalFilterUpdateStatus=on
  CAN Unpack2 : canmsglib/CAN Unpack  CANdbFile=C:\Users\EcoCAR_HIL\Documents\Khanna\EcoSIM3_P1_0_PHEV_TCU\Final_DBC\20150828 RMS PM CAN DB.dbc  MsgList=M192_Command_Message  MsgName=M192_Command_Message  MsgIDType=Standard (11-bit identifier)  MsgIdentifier=192  MsgLength=8  SignalInfo=Direction_Command$42$1$1$2$1$0$1$0$0$1$#Inverter_Discharge$41$1$1$2$1$0$1$0$0$1$#Inverter_Enable$40$1$1$2$1$0$1$0$0$1$#Speed_Command$16$16$1$1$1$0$1$0$-32768$32767$#Torque_Command$0$16$1$1$1$0$1.000000e-01$0$-3.276800e+03$3.276700e+03$#Torque_Limit_Command$48$16$1$1$1$0$1$0$-3.276800e+03$3.276700e+03$#  NSignals=6  IDPort=off  TimestampPort=off  ErrorPort=off  RemotePort=off  LengthPort=off  StatusPort=off  StartBits=str2num('[int32(42);int32(41);int32(40);int32(16);int32(0);int32(48)]')  SignalSizes=str2num('[int32(1);int32(1);int32(1);int32(16);int32(16);int32(16)]')  ByteOrders=str2num('[int32(1);int32(1);int32(1);int32(1);int32(1);int32(1)]')  DataTypes=str2num('[int32(2);int32(2);int32(2);int32(1);int32(1);int32(1)]')  MultiplexTypes=str2num('[int32(1);int32(1);int32(1);int32(1);int32(1);int32(1)]')  MultiplexValues=str2num('[double(0);double(0);double(0);double(0);double(0);double(0)]')  Factors=str2num('[double(1);double(1);double(1);double(1);double(1.000000e-01);double(1)]')  Offsets=str2num('[double(0);double(0);double(0);double(0);double(0);double(0)]')  Minimums=str2num('[double(0);double(0);double(0);double(-32768);double(-3.276800e+03);double(-3.276800e+03)]')  Maximums=str2num('[double(1);double(1);double(1);double(32767);double(3.276700e+03);double(3.276700e+03)]')
      settings: DataFormat=CANdb specified signals
  Terminator{5,7..9} (4 alike) : Terminator
  EM CAN : Outport
  wires:
  Bus Creator/1 -> EM CAN/1  "EM_CAN"
  Bus Creator1/1 -> Bus Creator/1  "M192_Command_Message"
  CAN Receive1/2 -> CAN Unpack2/1
  CAN Receive1/1 -> Terminator5/1
  CAN Unpack2/1 -> Bus Creator1/1  "Rotation_Direction"
  CAN Unpack2/3 -> Bus Creator1/2  "Inverter_Enable"
  CAN Unpack2/5 -> Bus Creator1/3  "Torque_Command"
  CAN Unpack2/2 -> Terminator7/1
  CAN Unpack2/4 -> Terminator8/1
  CAN Unpack2/6 -> Terminator9/1

== system EcoSIM3_P2_C2/Powertrain/Soft_ECUs_IO/VNT Kvaser/CANRx/ESS Receive ==
  Bus Creator5 : BusCreator
  Bus Creator6 : BusCreator  Inputs=1
  CAN Receive4 : canlib/CAN Receive  BlockHandle=2787.0027  DeviceMenu=Kvaser Virtual 1 (Channel 1)  Device=Kvaser Virtual 1 (Channel 1)  ObjConstructor=canChannel('Kvaser', 'Virtual 1', 1)  EnableStandardIDsFilter=off  StandardIDs=1024  EnableExtendedIDsFilter=off  ExtendedIDs=0  SampleTime=0.01  MsgsPerTimestep=1  StdIDsCombo=Allow only  ExtIDsCombo=Block all  InternalFilterUpdateStatus=on
  CAN Unpack4 : canmsglib/CAN Unpack  CANdbFile=C:\Users\EcoCAR_HIL\Documents\Khanna\EcoSIM3_P1_0_PHEV_TCU\Final_DBC\BCM_VehBus_Std.dbc  MsgList=BCM_Request  MsgName=BCM_Request  MsgIDType=Standard (11-bit identifier)  MsgIdentifier=1024  MsgLength=4  SignalInfo=hsc_bcm_enable$0$1$2$2$1$0$1$0$0$1$#hsc_bcm_epo$1$1$2$2$1$0$1$0$0$1$#hsc_bcm_leakage_ena$3$1$2$2$1$0$1$0$0$1$#hsc_bcm_mainc_close$2$1$2$2$1$0$1$0$0$1$#  NSignals=4  IDPort=off  TimestampPort=off  ErrorPort=off  RemotePort=off  LengthPort=off  StatusPort=off  StartBits=str2num('[int32(0);int32(1);int32(3);int32(2)]')  SignalSizes=str2num('[int32(1);int32(1);int32(1);int32(1)]')  ByteOrders=str2num('[int32(2);int32(2);int32(2);int32(2)]')  DataTypes=str2num('[int32(2);int32(2);int32(2);int32(2)]')  MultiplexTypes=str2num('[int32(1);int32(1);int32(1);int32(1)]')  MultiplexValues=str2num('[double(0);double(0);double(0);double(0)]')  Factors=str2num('[double(1);double(1);double(1);double(1)]')  Offsets=str2num('[double(0);double(0);double(0);double(0)]')  Minimums=str2num('[double(0);double(0);double(0);double(0)]')  Maximums=str2num('[double(1);double(1);double(1);double(1)]')
      settings: DataFormat=CANdb specified signals
  Terminator3 : Terminator
  ESS CAN : Outport
  wires:
  Bus Creator5/1 -> Bus Creator6/1  "BCM_Request"
  Bus Creator6/1 -> ESS CAN/1  "BCM_CAN"
  CAN Receive4/2 -> CAN Unpack4/1
  CAN Receive4/1 -> Terminator3/1
  CAN Unpack4/1 -> Bus Creator5/1  "hsc_bcm_enable"
  CAN Unpack4/2 -> Bus Creator5/2  "hsc_bcm_epo"
  CAN Unpack4/4 -> Bus Creator5/4  "hsc_bcm_mainc_close"
  CAN Unpack4/3 -> Bus Creator5/3  "hsc_bcm_leakage_ena"

== system EcoSIM3_P2_C2/Powertrain/Soft_ECUs_IO/VNT Kvaser/CANRx/ICE Receive ==
  Bus Creator14 : BusCreator  Inputs=1
  Bus Creator15 : BusCreator  Inputs=1
  CAN Receive2 : canlib/CAN Receive  BlockHandle=2802.0027  DeviceMenu=Kvaser Virtual 1 (Channel 1)  Device=Kvaser Virtual 1 (Channel 1)  ObjConstructor=canChannel('Kvaser', 'Virtual 1', 1)  EnableStandardIDsFilter=off  StandardIDs=101  EnableExtendedIDsFilter=off  ExtendedIDs=0  SampleTime=0.01  MsgsPerTimestep=1  StdIDsCombo=Allow only  ExtIDsCombo=Block all  InternalFilterUpdateStatus=on
  CAN Unpack1 : canmsglib/CAN Unpack  CANdbFile=C:\Users\EcoCAR_HIL\Documents\Khanna\EcoSIM3_P1_0_PHEV_TCU\Final_DBC\Engine_Transmission_BAS.dbc  MsgList=ECO_Engine_MSG101  MsgName=ECO_Engine_MSG101  MsgIDType=Standard (11-bit identifier)  MsgIdentifier=101  MsgLength=2  SignalInfo=ICE_Torque_Request_Nm$9$15$2$2$1$0$1.000000e-02$0$0$3.276700e+02$#  NSignals=1  IDPort=off  TimestampPort=off  ErrorPort=off  RemotePort=off  LengthPort=off  StatusPort=off  StartBits=str2num('[int32(9)]')  SignalSizes=str2num('[int32(15)]')  ByteOrders=str2num('[int32(2)]')  DataTypes=str2num('[int32(2)]')  MultiplexTypes=str2num('[int32(1)]')  MultiplexValues=str2num('[double(0)]')  Factors=str2num('[double(1.000000e-02)]')  Offsets=str2num('[double(0)]')  Minimums=str2num('[double(0)]')  Maximums=str2num('[double(3.276700e+02)]')
      settings: DataFormat=CANdb specified signals
  Terminator11 : Terminator
  ICE CAN : Outport
  wires:
  Bus Creator15/1 -> ICE CAN/1  "ICE_CAN"
  Bus Creator14/1 -> Bus Creator15/1  "ICE_Request"
  CAN Unpack1/1 -> Bus Creator14/1  "ICE_Torque_Request_Nm"
  CAN Receive2/2 -> CAN Unpack1/1
  CAN Receive2/1 -> Terminator11/1

== system EcoSIM3_P2_C2/Powertrain/Soft_ECUs_IO/VNT Kvaser/CANRx/Transmisssion Receive ==
  Bus Creator : BusCreator  Inputs=2
  Bus Creator18 : BusCreator  Inputs=1
  Bus Creator2 : BusCreator  Inputs=1
  CAN Receive1 : canlib/CAN Receive  BlockHandle=2815.0027  DeviceMenu=Kvaser Virtual 1 (Channel 1)  Device=Kvaser Virtual 1 (Channel 1)  ObjConstructor=canChannel('Kvaser', 'Virtual 1', 1)  EnableStandardIDsFilter=off  StandardIDs=94  EnableExtendedIDsFilter=off  ExtendedIDs=0  SampleTime=0.01  MsgsPerTimestep=1  StdIDsCombo=Allow only  ExtIDsCombo=Block all  InternalFilterUpdateStatus=on
  CAN Receive3 : canlib/CAN Receive  BlockHandle=2816.0023  DeviceMenu=Kvaser Virtual 1 (Channel 1)  Device=Kvaser Virtual 1 (Channel 1)  ObjConstructor=canChannel('Kvaser', 'Virtual 1', 1)  EnableStandardIDsFilter=off  StandardIDs=105  EnableExtendedIDsFilter=off  ExtendedIDs=0  SampleTime=0.01  MsgsPerTimestep=1  StdIDsCombo=Allow only  ExtIDsCombo=Block all  InternalFilterUpdateStatus=on
  CAN Unpack3 : canmsglib/CAN Unpack  CANdbFile=C:\Users\EcoCAR_HIL\Documents\Khanna\EcoSIM3_P1_0_PHEV_TCU\Final_DBC\Engine_Transmission_BAS.dbc  MsgList=ECO_Trans_Receive_MSG105  MsgName=ECO_Trans_Receive_MSG105  MsgIDType=Standard (11-bit identifier)  MsgIdentifier=105  MsgLength=1  SignalInfo=Clutch_Request$4$1$2$2$1$0$1$0$0$1$#Gear_Request$5$3$2$2$1$0$1$0$0$7$#  NSignals=2  IDPort=off  TimestampPort=off  ErrorPort=off  RemotePort=off  LengthPort=off  StatusPort=off  StartBits=str2num('[int32(4);int32(5)]')  SignalSizes=str2num('[int32(1);int32(3)]')  ByteOrders=str2num('[int32(2);int32(2)]')  DataTypes=str2num('[int32(2);int32(2)]')  MultiplexTypes=str2num('[int32(1);int32(1)]')  MultiplexValues=str2num('[double(0);double(0)]')  Factors=str2num('[double(1);double(1)]')  Offsets=str2num('[double(0);double(0)]')  Minimums=str2num('[double(0);double(0)]')  Maximums=str2num('[double(1);double(7)]')
      settings: DataFormat=CANdb specified signals
  CAN Unpack5 : canmsglib/CAN Unpack  CANdbFile=C:\Users\EcoCAR_HIL\Documents\Khanna\EcoSIM3_P1_0_PHEV_TCU\Final_DBC\EcoCAR3_Controls_Development.dbc  MsgList=MABx_Transmit_MSG094  MsgName=MABx_Transmit_MSG094  MsgIDType=Standard (11-bit identifier)  MsgIdentifier=94  MsgLength=1  SignalInfo=Mode$7$1$2$2$1$0$1$0$0$1$#  NSignals=1  IDPort=off  TimestampPort=off  ErrorPort=off  RemotePort=off  LengthPort=off  StatusPort=off  StartBits=str2num('[int32(7)]')  SignalSizes=str2num('[int32(1)]')  ByteOrders=str2num('[int32(2)]')  DataTypes=str2num('[int32(2)]')  MultiplexTypes=str2num('[int32(1)]')  MultiplexValues=str2num('[double(0)]')  Factors=str2num('[double(1)]')  Offsets=str2num('[double(0)]')  Minimums=str2num('[double(0)]')  Maximums=str2num('[double(1)]')
      settings: DataFormat=CANdb specified signals
  Ground : Ground
  Terminator1 : Terminator
  Terminator12 : Terminator
  Terminator13 : Terminator
  Clutch_Trans : Outport
  Mode : Outport  Port=2
  wires:
  Bus Creator18/1 -> Clutch_Trans/1  "Clutch_Trans_CAN"
  Bus Creator/1 -> Mode/1  "Supervisory"
  CAN Unpack5/1 -> Bus Creator/1  "Mode"
  Ground/1 -> Bus Creator/2  "Driver Torque Request"
  CAN Receive3/1 -> Terminator12/1
  Bus Creator2/1 -> Bus Creator18/1  "Trans_Receive"
  CAN Receive3/2 -> CAN Unpack3/1
  CAN Unpack3/2 -> Bus Creator2/1  "Gear_Request"
  CAN Unpack3/1 -> Terminator13/1  "Clutch_Request"
  CAN Receive1/1 -> Terminator1/1
  CAN Receive1/2 -> CAN Unpack5/1

== system EcoSIM3_P2_C2/Powertrain/Soft_ECUs_IO/VNT Kvaser/CANTx/BAS ==
  BAS : Inport
  Bus Selector5 : BusSelector  OutputSignals=Status_1.BAS_Speed_rad_per_s,Status_1.BAS_Torque_Out_Nm,Status_2.Fault_U,Status_2.Fault_V,Status_2.Fault_W
  CAN Pack5 : canmsglib/CAN Pack  CANdbFile=C:\Users\EcoCAR_HIL\Documents\Khanna\EcoSIM3_P1_0_PHEV_TCU\Final_DBC\Engine_Transmission_BAS.dbc  MsgList=ECO_BAS_Status_MSG099  MsgName=ECO_BAS_Status_MSG099  MsgIDType=Standard (11-bit identifier)  MsgIdentifier=99  MsgLength=5  SignalInfo=BAS_Fault_Status$36$1$2$2$1$0$1$0$0$1$#BAS_Speed_rad_per_s$8$16$2$1$1$0$1.000000e-01$0$-3.276800e+03$3.276700e+03$#BAS_Status_Mode$37$1$2$2$1$0$1$0$0$1$#BAS_Torque_Command_Nm$25$15$2$1$1$0$1.000000e-02$0$-1.638400e+02$1.638300e+02$#Fault_U$24$1$2$2$1$0$1$0$0$1$#Fault_V$39$1$2$2$1$0$1$0$0$1$#Fault_W$38$1$2$2$1$0$1$0$0$1$#  NSignals=7  StartBits=str2num('[int32(36);int32(8);int32(37);int32(25);int32(24);int32(39);int32(38)]')  SignalSizes=str2num('[int32(1);int32(16);int32(1);int32(15);int32(1);int32(1);int32(1)]')  ByteOrders=str2num('[int32(2);int32(2);int32(2);int32(2);int32(2);int32(2);int32(2)]')  DataTypes=str2num('[int32(2);int32(1);int32(2);int32(1);int32(2);int32(2);int32(2)]')  MultiplexTypes=str2num('[int32(1);int32(1);int32(1);int32(1);int32(1);int32(1);int32(1)]')  MultiplexValues=str2num('[double(0);double(0);double(0);double(0);double(0);double(0);double(0)]')  Factors=str2num('[double(1);double(1.000000e-01);double(1);double(1.000000e-02);double(1);double(1);double(1)]')  Offsets=str2num('[double(0);double(0);double(0);double(0);double(0);double(0);double(0)]')  Minimums=str2num('[double(0);double(-3.276800e+03);double(0);double(-1.638400e+02);double(0);double(0);double(0)]')  Maximums=str2num('[double(1);double(3.276700e+03);double(1);double(1.638300e+02);double(1);double(1);double(1)]')  Remote=off
      settings: DataFormat=CANdb specified signals
  CAN Transmit5 : canlib/CAN Transmit  BlockHandle=2851.0023  DeviceMenu=Kvaser Virtual 1 (Channel 1)  Device=Kvaser Virtual 1 (Channel 1)  ObjConstructor=canChannel('Kvaser', 'Virtual 1', 1)  EnablePeriodicTransmit=off  MessagePeriod=1.000
  Ground_1 : Ground
  Ground_2 : Ground
  wires:
  Ground_2/1 -> CAN Pack5/3
  Ground_1/1 -> CAN Pack5/1
  Bus Selector5/5 -> CAN Pack5/7  "<Fault_W>"
  Bus Selector5/4 -> CAN Pack5/6  "<Fault_V>"
  Bus Selector5/3 -> CAN Pack5/5  "<Fault_U>"
  Bus Selector5/2 -> CAN Pack5/4  "<BAS_Torque_Out_Nm>"
  Bus Selector5/1 -> CAN Pack5/2  "<BAS_Speed_rad_per_s>"
  BAS/1 -> Bus Selector5/1
  CAN Pack5/1 -> CAN Transmit5/1

== system EcoSIM3_P2_C2/Powertrain/Soft_ECUs_IO/VNT Kvaser/CANTx/Brusa ==
  Brusa : Inport
  Bus Selector5 : BusSelector  OutputSignals=Brusa_Dummy_msg.Dummy1,Brusa_Dummy_msg.Dummy2
  Terminator : Terminator
  Terminator1 : Terminator
  wires:
  Brusa/1 -> Bus Selector5/1
  Bus Selector5/1 -> Terminator/1  "<Dummy1>"
  Bus Selector5/2 -> Terminator1/1  "<Dummy2>"

== system EcoSIM3_P2_C2/Powertrain/Soft_ECUs_IO/VNT Kvaser/CANTx/Clutch_and_Trans ==
  Trans : Inport
  Bus Selector4 : BusSelector  OutputSignals=Message_1.Actual_Gear
  CAN Pack3 : canmsglib/CAN Pack  CANdbFile=C:\Users\EcoCAR_HIL\Documents\Khanna\EcoSIM3_P1_0_PHEV_TCU\Final_DBC\Engine_Transmission_BAS.dbc  MsgList=ECO_Trans_Status_MSG106  MsgName=ECO_Trans_Status_MSG106  MsgIDType=Standard (11-bit identifier)  MsgIdentifier=106  MsgLength=1  SignalInfo=Actual_Gear$1$3$2$2$1$0$1$0$0$7$#Clutch_Sw$7$1$2$2$1$0$1$0$0$1$#TCM_Gear$4$3$2$2$1$0$1$0$0$7$#  NSignals=3  StartBits=str2num('[int32(1);int32(7);int32(4)]')  SignalSizes=str2num('[int32(3);int32(1);int32(3)]')  ByteOrders=str2num('[int32(2);int32(2);int32(2)]')  DataTypes=str2num('[int32(2);int32(2);int32(2)]')  MultiplexTypes=str2num('[int32(1);int32(1);int32(1)]')  MultiplexValues=str2num('[double(0);double(0);double(0)]')  Factors=str2num('[double(1);double(1);double(1)]')  Offsets=str2num('[double(0);double(0);double(0)]')  Minimums=str2num('[double(0);double(0);double(0)]')  Maximums=str2num('[double(7);double(1);double(7)]')  Remote=off
      settings: DataFormat=CANdb specified signals
  CAN Transmit3 : canlib/CAN Transmit  BlockHandle=2876.0023  DeviceMenu=Kvaser Virtual 1 (Channel 1)  Device=Kvaser Virtual 1 (Channel 1)  ObjConstructor=canChannel('Kvaser', 'Virtual 1', 1)  EnablePeriodicTransmit=off  MessagePeriod=1.000
  Ground10 : Ground
  Ground11 : Ground
  wires:
  Ground11/1 -> CAN Pack3/3
  Ground10/1 -> CAN Pack3/2
  Bus Selector4/1 -> CAN Pack3/1  "<Actual_Gear>"
  CAN Pack3/1 -> CAN Transmit3/1
  Trans/1 -> Bus Selector4/1

== system EcoSIM3_P2_C2/Powertrain/Soft_ECUs_IO/VNT Kvaser/CANTx/EM ==
  EM : Inport
  M160_Temperature_Set_1 : Subsystem
  M161_Temperature_Set_2 : Subsystem
  M162_Temperature_Set_3 : Subsystem
  M165_Motor_Position_Info : Subsystem
  M170_Internal_States : Subsystem
  M171_Fault_Codes : Subsystem
  M172_Torque_And_Timer_Info : Subsystem
  wires:
  EM/1 -> M160_Temperature_Set_1/1(EM), M161_Temperature_Set_2/1(EM), M162_Temperature_Set_3/1(EM), M170_Internal_States/1(EM), M172_Torque_And_Timer_Info/1(EM), M165_Motor_Position_Info/1(EM), M171_Fault_Codes/1(EM)

== system EcoSIM3_P2_C2/Powertrain/Soft_ECUs_IO/VNT Kvaser/CANTx/ESS ==
  ESS : Inport
  BCM_Data : Subsystem
  BCM_Limits : Subsystem
  BCM_Status : Subsystem
  wires:
  ESS/1 -> BCM_Data/1(ESS), BCM_Status/1(ESS), BCM_Limits/1(ESS)

== system EcoSIM3_P2_C2/Powertrain/Soft_ECUs_IO/VNT Kvaser/CANTx/Engine ==
  ICE : Inport
  Bus Selector1 : BusSelector  OutputSignals=ICE_Torque.ICE_Torque_Cmd_Nm
  CAN Pack : canmsglib/CAN Pack  CANdbFile=C:\Users\EcoCAR_HIL\Documents\Khanna\EcoSIM3_P1_0_PHEV_TCU\Final_DBC\Engine_Transmission_BAS.dbc  MsgList=ECO_Engine_MSG104  MsgName=ECO_Engine_MSG104  MsgIDType=Standard (11-bit identifier)  MsgIdentifier=104  MsgLength=2  SignalInfo=ICE_Torque_Cmd_Nm$9$15$2$2$1$0$1.000000e-02$0$0$3.276700e+02$#  NSignals=1  StartBits=str2num('[int32(9)]')  SignalSizes=str2num('[int32(15)]')  ByteOrders=str2num('[int32(2)]')  DataTypes=str2num('[int32(2)]')  MultiplexTypes=str2num('[int32(1)]')  MultiplexValues=str2num('[double(0)]')  Factors=str2num('[double(1.000000e-02)]')  Offsets=str2num('[double(0)]')  Minimums=str2num('[double(0)]')  Maximums=str2num('[double(3.276700e+02)]')  Remote=off
      settings: DataFormat=CANdb specified signals
  CAN Transmit : canlib/CAN Transmit  BlockHandle=3132.0018  DeviceMenu=Kvaser Virtual 1 (Channel 1)  Device=Kvaser Virtual 1 (Channel 1)  ObjConstructor=canChannel('Kvaser', 'Virtual 1', 1)  EnablePeriodicTransmit=off  MessagePeriod=1.000
  wires:
  CAN Pack/1 -> CAN Transmit/1
  Bus Selector1/1 -> CAN Pack/1  "<ICE_Torque_Cmd_Nm>"
  ICE/1 -> Bus Selector1/1

== system EcoSIM3_P2_C2/Powertrain/Soft_ECUs_IO/VNT Kvaser/CANTx/GMLAN ==
  Driver : Inport
  PPEI_Brake_Apply_Status : Subsystem
  PPEI_Driven_Whl_Rotational_Stat : Subsystem
  PPEI_NonDrivn_Whl_Rotationl_Stat : Subsystem
  PPEI_Platform_General_Status : Subsystem
  PPEI_Vehicle_Speed_and_Distance : Subsystem
  wires:
  Driver/1 -> PPEI_Vehicle_Speed_and_Distance/1(GM), PPEI_NonDrivn_Whl_Rotationl_Stat/1(GM), PPEI_Driven_Whl_Rotational_Stat/1(GM), PPEI_Platform_General_Status/1(GM), PPEI_Brake_Apply_Status/1(GM)
